simulink model "sparam_amp"  (Simulink 6.0)
settings: Solver=ode45  StartTime=0.0  StopTime=10  RelTol=1e-3
undefined symbols (not defined in the file or in its folder): Fs, read, rfdata
libraries: rfports1 x2, rfamplifiers1 x1, simulink x1, dspsnks4 x1, dspsrcs4 x1
settings Model: Creator=mikem  LastModifiedBy=rzeng  ProdHWDeviceType=Specified
settings DataIOCC: SaveOutput=off  SaveTime=off  SignalLoggingName=sigsOut
settings DebuggingCC: CheckExecutionContextPreStartOutputMsg=on  CheckExecutionContextRuntimeOutputMsg=on  SolverPrmCheckMsg=none
settings HardwareCC: ProdHWDeviceType=Specified
settings ModelReferenceCC: UpdateModelReferenceTargets=IfOutOfDate
settings SFSimCC: SFSimApplyToAllLibs=on  SFSimBuildMode=Incremental

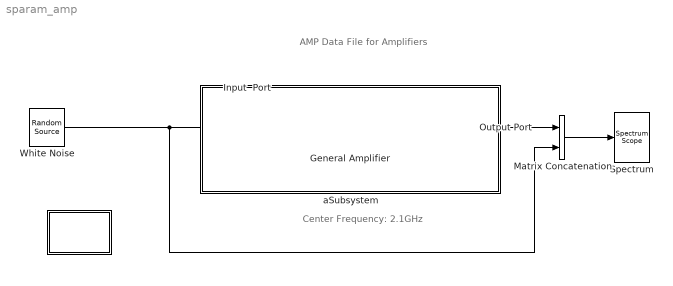
== system sparam_amp ==
  note: AMP Data File for Amplifiers
  note: Center Frequency: 2.1GHz
  " " : Subsystem  PropExecContextAcrossSSBoundary=on
      mask Type: Interpolation filter info block
      mask Display: disp('Info')
  General Amplifier : rfamplifiers1/General Amplifier  PhysicalDomain=rfsystemsdomain  SubClassName=general-amplifier  LeftPortType=p1  RightPortType=p1  LConnTagsString=__newl0  RConnTagsString=__newr0  RFDATA=read(rfdata.data, 'default.amp')  InterpMethod=Linear  IP3Type=OIP3  IIP3=inf  OIP3=inf  NF=0  DisplayData=off  PlotFreq=Derived from Input Port parameters  PlotFreqNoSim=Extracted from RFDATA object  Freq=[1.0e9:1.0e8:2.9e9]  AllPlotType=X-Y plane  NetworkData=S21  PowerData=S11  SmithData=S11  PolarData=S11  ComplexFormat=Magnitude (decibels)  DBFormat=Magnitude (decibels)  PowerFormat=dBm  PhaseFormat=Angle (degrees)  NoneFormat=None
  Input  Port : rfports1/Input Port  Description=source block  MaxLength=128  Fc=2.1e9  Ts=2e-9  Zs=50  NoiseFlag=off  seed=67987  GoToTag=BCDEKMGIUVAUFKJDKLBRSTA
  Matrix Concatenation : simulink/Math Operations/Matrix Concatenation  numInports=2  catMethod=Horizontal
  Output Port : rfports1/Output Port  Zl=50  num_Models=3  GoToTag=BCDEKMGIUVAUFKJDKLBRSTA  DisplayData=off  PlotFreq=Derived from Input Port parameters  Freq=1e9:1e8:3e9  AllPlotType=Composite data  NoBudgetPlot=Composite data  NetworkData=S11  SmithData=S11  PolarData=S11  ComplexFormat=Magnitude (decibels)  DBFormat=Magnitude (decibels)  DBMFormat=dBm  NoneFormat=None
  Spectrum : dspsnks4/Spectrum Scope  ScopeProperties=off  Domain=Frequency  HorizSpan=1  UseBuffer=on  BufferSize=1024  Overlap=512  inpFftLenInherit=on  FFTlength=1024  numAvg=100  DisplayProperties=on  AxisGrid=on  Memory=off  FrameNumber=on  AxisLegend=off  AxisZoom=off  OpenScopeAtSimStart=on  OpenScopeImmediately=off  FigPos=[5 288 399 283]  AxisProperties=off  XUnits=Hertz  XRange=[-Fs/2...Fs/2]  InheritXIncr=on  XIncr=1.0  XLabel=Samples  YUnits=dB  YLabel=Magnitude, dB  LineProperties=off  LineStyles=--  LineColors=|[1 0 0]
      settings: YMin=-5.86282795057197  YMax=17.1838347750497
  White Noise : dspsrcs4/Random Source  SrcType=Gaussian  NormMethod=Ziggurat  CltLength=12  Min=-1  Max=1  Mean=0  Var=1  RepMode=Not repeatable  rawSeed=1  Inherit=off  SampMode=Discrete  SampTime=2e-9  SampFrame=256  DataType=Double  OutComplex=Complex
  aSubsystem : Subsystem  PropExecContextAcrossSSBoundary=on
      mask Display: disp('')
  wires:
  Output Port/1 -> Matrix Concatenation/1
  White Noise/1 -> Input  Port/1, Matrix Concatenation/2
  Matrix Concatenation/1 -> Spectrum/1
  connections:
  Input  Port/RConn1 -- General Amplifier/LConn1
  General Amplifier/RConn1 -- Output Port/LConn1

== system sparam_amp/  ==
  note: AMP Data File for Amplifiers
      |
      | The Amplifiers library has blocks to handle
      | S, Y, and Z parameters of the amplifiers.
      | The library also has 'General Amplifier' block
      | that can be used for the AMP data file.
      |
      | The data file: 'default.amp' has
      | the S-parameters of an amplifier
      | over the frequency range 1GHz to 2.9GHz,
      | and Pin-Pot data at 2.1GHz.
      | The spectrum plot shows frequency ranging from
      | 1.85GHz to 2.35GHz centered at 2.1GHz.
      |
      | If you want to see the frequency response centered at other RF frequency,
      | you need to change the Center frequency parameter in the
      | 'Input Port' block.
      |
      | If you want to change the range of frequency response that is determined by
      | the Sample time parameter specified in the 'Input Port' and 'White Noise' blocks,
      | you need to change the Sample time parameter in both blocks.

== system sparam_amp/aSubsystem ==
